simulink model "DV3A_String1_Diode"  (R2023b)
settings: Solver=VariableStepAuto  StartTime=0.0  StopTime=1  FixedStep=Ts_Power  MinStep=0.0025  RelTol=1e-4
PreLoadFcn:
  | Ts_Power=5e-4;
  | Slope_Vdc=1;
InitFcn:
  | Ts_Power=50e-6;
  | Tc=1e-5;%break algebraic loop time constant
StopFcn:
  | if exist('I','var') && exist('V','var')
  |    figure(1)
  |    clf
  |    n=find(I>=0);
  |    n=n(end);
  |    Vglobal=V(1:n);
  |    Iglobal=I(1:n);
  | 
  | 
  |    Pglobal=Vglobal.*Iglobal;
  |    n=find(Pglobal==max(Pglobal));
  |    Pmax=Pglobal(n);
  |    Vmp=Vglobal(n);
  |    Imp=Iglobal(n);
  | 
  | 
  |    subplot(211)
  |    plot(Vglobal, Iglobal,Vmp,Imp,'or')
  |    ylabel('Current (A)')
  |    title(sprintf('Global I-V & P-V characteristics\n %s' ,ModuleName))
  | 
  | 
  |    subplot(212)
  |    plot(Vglobal, Pglobal,Vmp,Pmax,'or')
  |    ylabel('Power (W)')
  |    xlabel('Voltage (V)')
  | end
model workspace (MAT data in the model file):
  slope_Vdc = 3.0848387096
undefined symbols (not defined in the file): Slope_Vdc_string1
libraries: spsPVArrayLib x142, spsVariableResistorLib x142, spsDiodeLib x29, spsCurrentMeasurementLib x1, spsVoltageMeasurementLib x1, spsControlledVoltageSourceLib x1, simulink x1, spspowerguiLib x1
(part 2 of 8)

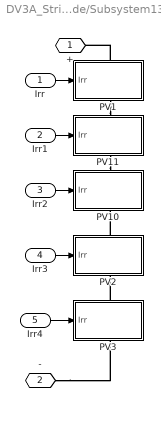
== system DV3A_String1_Diode/Subsystem13 ==
  Irr : Inport
  Irr1 : Inport  Port=2
  Irr2 : Inport  Port=3
  Irr3 : Inport  Port=4
  Irr4 : Inport  Port=5
  PV1 : Subsystem
      settings: PortSchema="{\"entries\":[{\"content\":{\"sides\":[{\"content\":{\"connectorIds\":[\"In1\"]},\"type\":\"ConnectorPlacement.EquallySpacedRectSide\",\"uuid\":\"5c508248-bd07-48d5-951d-be180bcc8740\"},{\"content\":{\"connectorIds\":[],\"side\":\"RIGHT\"},\"type\":\"ConnectorPlacement.EquallySpacedRectSide\",\"uuid\":\"e31a9bdc-b533-497f-8610-a92a4eef02bc\"},{\"content\":{\"connectorIds\":[\"LConn1\"],\"side\":\"TOP\"},\"type\":\"ConnectorPlacement.EquallySpacedRectSide\",\"uuid\":\"a80efd6c-0c74-41ec-a161-3d709011a457\"},{\"content\":{\"connectorIds\":[\"RConn1\"],\"side\":\"BOTTOM\"},\"type\":\"ConnectorPlacement.EquallySpacedRectSide\",\"uuid\":\"e2d028a7-872a-45fc-84e4-cb840db01281\"}]},\"type\":\"ConnectorPlacement.EquallySpacedConnector\",\"uuid\":\"57d442c0-d58c-4dd4-aeba-72d113e063d7\"}],\"packageUris\":[\"http://schema.mathworks.com/mf0/Connector/19700101\"],\"version\":\"1.0\"}"
  PV10 : Subsystem
      settings: PortSchema="{\"entries\":[{\"content\":{\"sides\":[{\"content\":{\"connectorIds\":[\"In1\"]},\"type\":\"ConnectorPlacement.EquallySpacedRectSide\",\"uuid\":\"5c508248-bd07-48d5-951d-be180bcc8740\"},{\"content\":{\"connectorIds\":[],\"side\":\"RIGHT\"},\"type\":\"ConnectorPlacement.EquallySpacedRectSide\",\"uuid\":\"e31a9bdc-b533-497f-8610-a92a4eef02bc\"},{\"content\":{\"connectorIds\":[\"LConn1\"],\"side\":\"TOP\"},\"type\":\"ConnectorPlacement.EquallySpacedRectSide\",\"uuid\":\"a80efd6c-0c74-41ec-a161-3d709011a457\"},{\"content\":{\"connectorIds\":[\"RConn1\"],\"side\":\"BOTTOM\"},\"type\":\"ConnectorPlacement.EquallySpacedRectSide\",\"uuid\":\"e2d028a7-872a-45fc-84e4-cb840db01281\"}]},\"type\":\"ConnectorPlacement.EquallySpacedConnector\",\"uuid\":\"57d442c0-d58c-4dd4-aeba-72d113e063d7\"}],\"packageUris\":[\"http://schema.mathworks.com/mf0/Connector/19700101\"],\"version\":\"1.0\"}"
  PV11 : Subsystem
      settings: PortSchema="{\"entries\":[{\"content\":{\"sides\":[{\"content\":{\"connectorIds\":[\"In1\"]},\"type\":\"ConnectorPlacement.EquallySpacedRectSide\",\"uuid\":\"5c508248-bd07-48d5-951d-be180bcc8740\"},{\"content\":{\"connectorIds\":[],\"side\":\"RIGHT\"},\"type\":\"ConnectorPlacement.EquallySpacedRectSide\",\"uuid\":\"e31a9bdc-b533-497f-8610-a92a4eef02bc\"},{\"content\":{\"connectorIds\":[\"LConn1\"],\"side\":\"TOP\"},\"type\":\"ConnectorPlacement.EquallySpacedRectSide\",\"uuid\":\"a80efd6c-0c74-41ec-a161-3d709011a457\"},{\"content\":{\"connectorIds\":[\"RConn1\"],\"side\":\"BOTTOM\"},\"type\":\"ConnectorPlacement.EquallySpacedRectSide\",\"uuid\":\"e2d028a7-872a-45fc-84e4-cb840db01281\"}]},\"type\":\"ConnectorPlacement.EquallySpacedConnector\",\"uuid\":\"57d442c0-d58c-4dd4-aeba-72d113e063d7\"}],\"packageUris\":[\"http://schema.mathworks.com/mf0/Connector/19700101\"],\"version\":\"1.0\"}"
  PV2 : Subsystem
      settings: PortSchema="{\"entries\":[{\"content\":{\"sides\":[{\"content\":{\"connectorIds\":[\"In1\"]},\"type\":\"ConnectorPlacement.EquallySpacedRectSide\",\"uuid\":\"5c508248-bd07-48d5-951d-be180bcc8740\"},{\"content\":{\"connectorIds\":[],\"side\":\"RIGHT\"},\"type\":\"ConnectorPlacement.EquallySpacedRectSide\",\"uuid\":\"e31a9bdc-b533-497f-8610-a92a4eef02bc\"},{\"content\":{\"connectorIds\":[\"LConn1\"],\"side\":\"TOP\"},\"type\":\"ConnectorPlacement.EquallySpacedRectSide\",\"uuid\":\"a80efd6c-0c74-41ec-a161-3d709011a457\"},{\"content\":{\"connectorIds\":[\"RConn1\"],\"side\":\"BOTTOM\"},\"type\":\"ConnectorPlacement.EquallySpacedRectSide\",\"uuid\":\"e2d028a7-872a-45fc-84e4-cb840db01281\"}]},\"type\":\"ConnectorPlacement.EquallySpacedConnector\",\"uuid\":\"57d442c0-d58c-4dd4-aeba-72d113e063d7\"}],\"packageUris\":[\"http://schema.mathworks.com/mf0/Connector/19700101\"],\"version\":\"1.0\"}"
  PV3 : Subsystem
      settings: PortSchema="{\"entries\":[{\"content\":{\"sides\":[{\"content\":{\"connectorIds\":[\"In1\"]},\"type\":\"ConnectorPlacement.EquallySpacedRectSide\",\"uuid\":\"5c508248-bd07-48d5-951d-be180bcc8740\"},{\"content\":{\"connectorIds\":[],\"side\":\"RIGHT\"},\"type\":\"ConnectorPlacement.EquallySpacedRectSide\",\"uuid\":\"e31a9bdc-b533-497f-8610-a92a4eef02bc\"},{\"content\":{\"connectorIds\":[\"LConn1\"],\"side\":\"TOP\"},\"type\":\"ConnectorPlacement.EquallySpacedRectSide\",\"uuid\":\"a80efd6c-0c74-41ec-a161-3d709011a457\"},{\"content\":{\"connectorIds\":[\"RConn1\"],\"side\":\"BOTTOM\"},\"type\":\"ConnectorPlacement.EquallySpacedRectSide\",\"uuid\":\"e2d028a7-872a-45fc-84e4-cb840db01281\"}]},\"type\":\"ConnectorPlacement.EquallySpacedConnector\",\"uuid\":\"57d442c0-d58c-4dd4-aeba-72d113e063d7\"}],\"packageUris\":[\"http://schema.mathworks.com/mf0/Connector/19700101\"],\"version\":\"1.0\"}"
  + : PMIOPort  Side=Left
  - : PMIOPort  Port=2  Side=Right
  wires:
  Irr2/1 -> PV10/1(Irr)
  Irr/1 -> PV1/1(Irr)
  Irr1/1 -> PV11/1(Irr)
  Irr3/1 -> PV2/1(Irr)
  Irr4/1 -> PV3/1(Irr)
  connections:
  PV1/LConn1 -- +/RConn1
  PV11/RConn1 -- PV10/LConn1
  PV1/RConn1 -- PV11/LConn1
  PV2/LConn1 -- PV10/RConn1
  PV3/LConn1 -- PV2/RConn1
  -/RConn1 -- PV3/RConn1

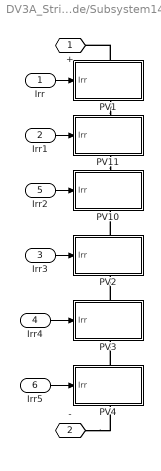
== system DV3A_String1_Diode/Subsystem14 ==
  Irr : Inport
  Irr1 : Inport  Port=2
  Irr3 : Inport  Port=3
  Irr4 : Inport  Port=4
  Irr2 : Inport  Port=5
  Irr5 : Inport  Port=6
  PV1 : Subsystem
      settings: PortSchema="{\"entries\":[{\"content\":{\"sides\":[{\"content\":{\"connectorIds\":[\"In1\"]},\"type\":\"ConnectorPlacement.EquallySpacedRectSide\",\"uuid\":\"5c508248-bd07-48d5-951d-be180bcc8740\"},{\"content\":{\"connectorIds\":[],\"side\":\"RIGHT\"},\"type\":\"ConnectorPlacement.EquallySpacedRectSide\",\"uuid\":\"e31a9bdc-b533-497f-8610-a92a4eef02bc\"},{\"content\":{\"connectorIds\":[\"LConn1\"],\"side\":\"TOP\"},\"type\":\"ConnectorPlacement.EquallySpacedRectSide\",\"uuid\":\"a80efd6c-0c74-41ec-a161-3d709011a457\"},{\"content\":{\"connectorIds\":[\"RConn1\"],\"side\":\"BOTTOM\"},\"type\":\"ConnectorPlacement.EquallySpacedRectSide\",\"uuid\":\"e2d028a7-872a-45fc-84e4-cb840db01281\"}]},\"type\":\"ConnectorPlacement.EquallySpacedConnector\",\"uuid\":\"57d442c0-d58c-4dd4-aeba-72d113e063d7\"}],\"packageUris\":[\"http://schema.mathworks.com/mf0/Connector/19700101\"],\"version\":\"1.0\"}"
  PV10 : Subsystem
      settings: PortSchema="{\"entries\":[{\"content\":{\"sides\":[{\"content\":{\"connectorIds\":[\"In1\"]},\"type\":\"ConnectorPlacement.EquallySpacedRectSide\",\"uuid\":\"5c508248-bd07-48d5-951d-be180bcc8740\"},{\"content\":{\"connectorIds\":[],\"side\":\"RIGHT\"},\"type\":\"ConnectorPlacement.EquallySpacedRectSide\",\"uuid\":\"e31a9bdc-b533-497f-8610-a92a4eef02bc\"},{\"content\":{\"connectorIds\":[\"LConn1\"],\"side\":\"TOP\"},\"type\":\"ConnectorPlacement.EquallySpacedRectSide\",\"uuid\":\"a80efd6c-0c74-41ec-a161-3d709011a457\"},{\"content\":{\"connectorIds\":[\"RConn1\"],\"side\":\"BOTTOM\"},\"type\":\"ConnectorPlacement.EquallySpacedRectSide\",\"uuid\":\"e2d028a7-872a-45fc-84e4-cb840db01281\"}]},\"type\":\"ConnectorPlacement.EquallySpacedConnector\",\"uuid\":\"57d442c0-d58c-4dd4-aeba-72d113e063d7\"}],\"packageUris\":[\"http://schema.mathworks.com/mf0/Connector/19700101\"],\"version\":\"1.0\"}"
  PV11 : Subsystem
      settings: PortSchema="{\"entries\":[{\"content\":{\"sides\":[{\"content\":{\"connectorIds\":[\"In1\"]},\"type\":\"ConnectorPlacement.EquallySpacedRectSide\",\"uuid\":\"5c508248-bd07-48d5-951d-be180bcc8740\"},{\"content\":{\"connectorIds\":[],\"side\":\"RIGHT\"},\"type\":\"ConnectorPlacement.EquallySpacedRectSide\",\"uuid\":\"e31a9bdc-b533-497f-8610-a92a4eef02bc\"},{\"content\":{\"connectorIds\":[\"LConn1\"],\"side\":\"TOP\"},\"type\":\"ConnectorPlacement.EquallySpacedRectSide\",\"uuid\":\"a80efd6c-0c74-41ec-a161-3d709011a457\"},{\"content\":{\"connectorIds\":[\"RConn1\"],\"side\":\"BOTTOM\"},\"type\":\"ConnectorPlacement.EquallySpacedRectSide\",\"uuid\":\"e2d028a7-872a-45fc-84e4-cb840db01281\"}]},\"type\":\"ConnectorPlacement.EquallySpacedConnector\",\"uuid\":\"57d442c0-d58c-4dd4-aeba-72d113e063d7\"}],\"packageUris\":[\"http://schema.mathworks.com/mf0/Connector/19700101\"],\"version\":\"1.0\"}"
  PV2 : Subsystem
      settings: PortSchema="{\"entries\":[{\"content\":{\"sides\":[{\"content\":{\"connectorIds\":[\"In1\"]},\"type\":\"ConnectorPlacement.EquallySpacedRectSide\",\"uuid\":\"5c508248-bd07-48d5-951d-be180bcc8740\"},{\"content\":{\"connectorIds\":[],\"side\":\"RIGHT\"},\"type\":\"ConnectorPlacement.EquallySpacedRectSide\",\"uuid\":\"e31a9bdc-b533-497f-8610-a92a4eef02bc\"},{\"content\":{\"connectorIds\":[\"LConn1\"],\"side\":\"TOP\"},\"type\":\"ConnectorPlacement.EquallySpacedRectSide\",\"uuid\":\"a80efd6c-0c74-41ec-a161-3d709011a457\"},{\"content\":{\"connectorIds\":[\"RConn1\"],\"side\":\"BOTTOM\"},\"type\":\"ConnectorPlacement.EquallySpacedRectSide\",\"uuid\":\"e2d028a7-872a-45fc-84e4-cb840db01281\"}]},\"type\":\"ConnectorPlacement.EquallySpacedConnector\",\"uuid\":\"57d442c0-d58c-4dd4-aeba-72d113e063d7\"}],\"packageUris\":[\"http://schema.mathworks.com/mf0/Connector/19700101\"],\"version\":\"1.0\"}"
  PV3 : Subsystem
      settings: PortSchema="{\"entries\":[{\"content\":{\"sides\":[{\"content\":{\"connectorIds\":[\"In1\"]},\"type\":\"ConnectorPlacement.EquallySpacedRectSide\",\"uuid\":\"5c508248-bd07-48d5-951d-be180bcc8740\"},{\"content\":{\"connectorIds\":[],\"side\":\"RIGHT\"},\"type\":\"ConnectorPlacement.EquallySpacedRectSide\",\"uuid\":\"e31a9bdc-b533-497f-8610-a92a4eef02bc\"},{\"content\":{\"connectorIds\":[\"LConn1\"],\"side\":\"TOP\"},\"type\":\"ConnectorPlacement.EquallySpacedRectSide\",\"uuid\":\"a80efd6c-0c74-41ec-a161-3d709011a457\"},{\"content\":{\"connectorIds\":[\"RConn1\"],\"side\":\"BOTTOM\"},\"type\":\"ConnectorPlacement.EquallySpacedRectSide\",\"uuid\":\"e2d028a7-872a-45fc-84e4-cb840db01281\"}]},\"type\":\"ConnectorPlacement.EquallySpacedConnector\",\"uuid\":\"57d442c0-d58c-4dd4-aeba-72d113e063d7\"}],\"packageUris\":[\"http://schema.mathworks.com/mf0/Connector/19700101\"],\"version\":\"1.0\"}"
  PV4 : Subsystem
      settings: PortSchema="{\"entries\":[{\"content\":{\"sides\":[{\"content\":{\"connectorIds\":[\"In1\"]},\"type\":\"ConnectorPlacement.EquallySpacedRectSide\",\"uuid\":\"5c508248-bd07-48d5-951d-be180bcc8740\"},{\"content\":{\"connectorIds\":[],\"side\":\"RIGHT\"},\"type\":\"ConnectorPlacement.EquallySpacedRectSide\",\"uuid\":\"e31a9bdc-b533-497f-8610-a92a4eef02bc\"},{\"content\":{\"connectorIds\":[\"LConn1\"],\"side\":\"TOP\"},\"type\":\"ConnectorPlacement.EquallySpacedRectSide\",\"uuid\":\"a80efd6c-0c74-41ec-a161-3d709011a457\"},{\"content\":{\"connectorIds\":[\"RConn1\"],\"side\":\"BOTTOM\"},\"type\":\"ConnectorPlacement.EquallySpacedRectSide\",\"uuid\":\"e2d028a7-872a-45fc-84e4-cb840db01281\"}]},\"type\":\"ConnectorPlacement.EquallySpacedConnector\",\"uuid\":\"57d442c0-d58c-4dd4-aeba-72d113e063d7\"}],\"packageUris\":[\"http://schema.mathworks.com/mf0/Connector/19700101\"],\"version\":\"1.0\"}"
  + : PMIOPort  Side=Left
  - : PMIOPort  Port=2  Side=Right
  wires:
  Irr2/1 -> PV10/1(Irr)
  Irr/1 -> PV1/1(Irr)
  Irr1/1 -> PV11/1(Irr)
  Irr3/1 -> PV2/1(Irr)
  Irr4/1 -> PV3/1(Irr)
  Irr5/1 -> PV4/1(Irr)
  connections:
  PV1/LConn1 -- +/RConn1
  PV11/RConn1 -- PV10/LConn1
  PV1/RConn1 -- PV11/LConn1
  PV2/LConn1 -- PV10/RConn1
  PV3/LConn1 -- PV2/RConn1
  PV4/LConn1 -- PV3/RConn1
  -/RConn1 -- PV4/RConn1

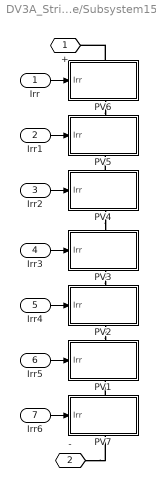
== system DV3A_String1_Diode/Subsystem15 ==
  Irr : Inport
  Irr1 : Inport  Port=2
  Irr2 : Inport  Port=3
  Irr3 : Inport  Port=4
  Irr4 : Inport  Port=5
  Irr5 : Inport  Port=6
  Irr6 : Inport  Port=7
  PV1 : Subsystem
      settings: PortSchema="{\"entries\":[{\"content\":{\"sides\":[{\"content\":{\"connectorIds\":[\"In1\"]},\"type\":\"ConnectorPlacement.EquallySpacedRectSide\",\"uuid\":\"5c508248-bd07-48d5-951d-be180bcc8740\"},{\"content\":{\"connectorIds\":[],\"side\":\"RIGHT\"},\"type\":\"ConnectorPlacement.EquallySpacedRectSide\",\"uuid\":\"e31a9bdc-b533-497f-8610-a92a4eef02bc\"},{\"content\":{\"connectorIds\":[\"LConn1\"],\"side\":\"TOP\"},\"type\":\"ConnectorPlacement.EquallySpacedRectSide\",\"uuid\":\"a80efd6c-0c74-41ec-a161-3d709011a457\"},{\"content\":{\"connectorIds\":[\"RConn1\"],\"side\":\"BOTTOM\"},\"type\":\"ConnectorPlacement.EquallySpacedRectSide\",\"uuid\":\"e2d028a7-872a-45fc-84e4-cb840db01281\"}]},\"type\":\"ConnectorPlacement.EquallySpacedConnector\",\"uuid\":\"57d442c0-d58c-4dd4-aeba-72d113e063d7\"}],\"packageUris\":[\"http://schema.mathworks.com/mf0/Connector/19700101\"],\"version\":\"1.0\"}"
  PV2 : Subsystem
      settings: PortSchema="{\"entries\":[{\"content\":{\"sides\":[{\"content\":{\"connectorIds\":[\"In1\"]},\"type\":\"ConnectorPlacement.EquallySpacedRectSide\",\"uuid\":\"5c508248-bd07-48d5-951d-be180bcc8740\"},{\"content\":{\"connectorIds\":[],\"side\":\"RIGHT\"},\"type\":\"ConnectorPlacement.EquallySpacedRectSide\",\"uuid\":\"e31a9bdc-b533-497f-8610-a92a4eef02bc\"},{\"content\":{\"connectorIds\":[\"LConn1\"],\"side\":\"TOP\"},\"type\":\"ConnectorPlacement.EquallySpacedRectSide\",\"uuid\":\"a80efd6c-0c74-41ec-a161-3d709011a457\"},{\"content\":{\"connectorIds\":[\"RConn1\"],\"side\":\"BOTTOM\"},\"type\":\"ConnectorPlacement.EquallySpacedRectSide\",\"uuid\":\"e2d028a7-872a-45fc-84e4-cb840db01281\"}]},\"type\":\"ConnectorPlacement.EquallySpacedConnector\",\"uuid\":\"57d442c0-d58c-4dd4-aeba-72d113e063d7\"}],\"packageUris\":[\"http://schema.mathworks.com/mf0/Connector/19700101\"],\"version\":\"1.0\"}"
  PV3 : Subsystem
      settings: PortSchema="{\"entries\":[{\"content\":{\"sides\":[{\"content\":{\"connectorIds\":[\"In1\"]},\"type\":\"ConnectorPlacement.EquallySpacedRectSide\",\"uuid\":\"5c508248-bd07-48d5-951d-be180bcc8740\"},{\"content\":{\"connectorIds\":[],\"side\":\"RIGHT\"},\"type\":\"ConnectorPlacement.EquallySpacedRectSide\",\"uuid\":\"e31a9bdc-b533-497f-8610-a92a4eef02bc\"},{\"content\":{\"connectorIds\":[\"LConn1\"],\"side\":\"TOP\"},\"type\":\"ConnectorPlacement.EquallySpacedRectSide\",\"uuid\":\"a80efd6c-0c74-41ec-a161-3d709011a457\"},{\"content\":{\"connectorIds\":[\"RConn1\"],\"side\":\"BOTTOM\"},\"type\":\"ConnectorPlacement.EquallySpacedRectSide\",\"uuid\":\"e2d028a7-872a-45fc-84e4-cb840db01281\"}]},\"type\":\"ConnectorPlacement.EquallySpacedConnector\",\"uuid\":\"57d442c0-d58c-4dd4-aeba-72d113e063d7\"}],\"packageUris\":[\"http://schema.mathworks.com/mf0/Connector/19700101\"],\"version\":\"1.0\"}"
  PV4 : Subsystem
      settings: PortSchema="{\"entries\":[{\"content\":{\"sides\":[{\"content\":{\"connectorIds\":[\"In1\"]},\"type\":\"ConnectorPlacement.EquallySpacedRectSide\",\"uuid\":\"5c508248-bd07-48d5-951d-be180bcc8740\"},{\"content\":{\"connectorIds\":[],\"side\":\"RIGHT\"},\"type\":\"ConnectorPlacement.EquallySpacedRectSide\",\"uuid\":\"e31a9bdc-b533-497f-8610-a92a4eef02bc\"},{\"content\":{\"connectorIds\":[\"LConn1\"],\"side\":\"TOP\"},\"type\":\"ConnectorPlacement.EquallySpacedRectSide\",\"uuid\":\"a80efd6c-0c74-41ec-a161-3d709011a457\"},{\"content\":{\"connectorIds\":[\"RConn1\"],\"side\":\"BOTTOM\"},\"type\":\"ConnectorPlacement.EquallySpacedRectSide\",\"uuid\":\"e2d028a7-872a-45fc-84e4-cb840db01281\"}]},\"type\":\"ConnectorPlacement.EquallySpacedConnector\",\"uuid\":\"57d442c0-d58c-4dd4-aeba-72d113e063d7\"}],\"packageUris\":[\"http://schema.mathworks.com/mf0/Connector/19700101\"],\"version\":\"1.0\"}"
  PV5 : Subsystem
      settings: PortSchema="{\"entries\":[{\"content\":{\"sides\":[{\"content\":{\"connectorIds\":[\"In1\"]},\"type\":\"ConnectorPlacement.EquallySpacedRectSide\",\"uuid\":\"5c508248-bd07-48d5-951d-be180bcc8740\"},{\"content\":{\"connectorIds\":[],\"side\":\"RIGHT\"},\"type\":\"ConnectorPlacement.EquallySpacedRectSide\",\"uuid\":\"e31a9bdc-b533-497f-8610-a92a4eef02bc\"},{\"content\":{\"connectorIds\":[\"LConn1\"],\"side\":\"TOP\"},\"type\":\"ConnectorPlacement.EquallySpacedRectSide\",\"uuid\":\"a80efd6c-0c74-41ec-a161-3d709011a457\"},{\"content\":{\"connectorIds\":[\"RConn1\"],\"side\":\"BOTTOM\"},\"type\":\"ConnectorPlacement.EquallySpacedRectSide\",\"uuid\":\"e2d028a7-872a-45fc-84e4-cb840db01281\"}]},\"type\":\"ConnectorPlacement.EquallySpacedConnector\",\"uuid\":\"57d442c0-d58c-4dd4-aeba-72d113e063d7\"}],\"packageUris\":[\"http://schema.mathworks.com/mf0/Connector/19700101\"],\"version\":\"1.0\"}"
  PV6 : Subsystem
      settings: PortSchema="{\"entries\":[{\"content\":{\"sides\":[{\"content\":{\"connectorIds\":[\"In1\"]},\"type\":\"ConnectorPlacement.EquallySpacedRectSide\",\"uuid\":\"5c508248-bd07-48d5-951d-be180bcc8740\"},{\"content\":{\"connectorIds\":[],\"side\":\"RIGHT\"},\"type\":\"ConnectorPlacement.EquallySpacedRectSide\",\"uuid\":\"e31a9bdc-b533-497f-8610-a92a4eef02bc\"},{\"content\":{\"connectorIds\":[\"LConn1\"],\"side\":\"TOP\"},\"type\":\"ConnectorPlacement.EquallySpacedRectSide\",\"uuid\":\"a80efd6c-0c74-41ec-a161-3d709011a457\"},{\"content\":{\"connectorIds\":[\"RConn1\"],\"side\":\"BOTTOM\"},\"type\":\"ConnectorPlacement.EquallySpacedRectSide\",\"uuid\":\"e2d028a7-872a-45fc-84e4-cb840db01281\"}]},\"type\":\"ConnectorPlacement.EquallySpacedConnector\",\"uuid\":\"57d442c0-d58c-4dd4-aeba-72d113e063d7\"}],\"packageUris\":[\"http://schema.mathworks.com/mf0/Connector/19700101\"],\"version\":\"1.0\"}"
  PV7 : Subsystem
      settings: PortSchema="{\"entries\":[{\"content\":{\"sides\":[{\"content\":{\"connectorIds\":[\"In1\"]},\"type\":\"ConnectorPlacement.EquallySpacedRectSide\",\"uuid\":\"5c508248-bd07-48d5-951d-be180bcc8740\"},{\"content\":{\"connectorIds\":[],\"side\":\"RIGHT\"},\"type\":\"ConnectorPlacement.EquallySpacedRectSide\",\"uuid\":\"e31a9bdc-b533-497f-8610-a92a4eef02bc\"},{\"content\":{\"connectorIds\":[\"LConn1\"],\"side\":\"TOP\"},\"type\":\"ConnectorPlacement.EquallySpacedRectSide\",\"uuid\":\"a80efd6c-0c74-41ec-a161-3d709011a457\"},{\"content\":{\"connectorIds\":[\"RConn1\"],\"side\":\"BOTTOM\"},\"type\":\"ConnectorPlacement.EquallySpacedRectSide\",\"uuid\":\"e2d028a7-872a-45fc-84e4-cb840db01281\"}]},\"type\":\"ConnectorPlacement.EquallySpacedConnector\",\"uuid\":\"57d442c0-d58c-4dd4-aeba-72d113e063d7\"}],\"packageUris\":[\"http://schema.mathworks.com/mf0/Connector/19700101\"],\"version\":\"1.0\"}"
  + : PMIOPort  Side=Left
  - : PMIOPort  Port=2  Side=Right
  wires:
  Irr2/1 -> PV4/1(Irr)
  Irr/1 -> PV6/1(Irr)
  Irr1/1 -> PV5/1(Irr)
  Irr3/1 -> PV3/1(Irr)
  Irr5/1 -> PV1/1(Irr)
  Irr4/1 -> PV2/1(Irr)
  Irr6/1 -> PV7/1(Irr)
  connections:
  PV6/LConn1 -- +/RConn1
  PV4/LConn1 -- PV5/RConn1
  PV6/RConn1 -- PV5/LConn1
  PV3/RConn1 -- PV2/LConn1
  PV2/RConn1 -- PV1/LConn1
  PV4/RConn1 -- PV3/LConn1
  -/RConn1 -- PV7/RConn1
  PV7/LConn1 -- PV1/RConn1

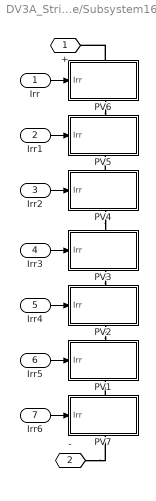
== system DV3A_String1_Diode/Subsystem16 ==
  Irr : Inport
  Irr1 : Inport  Port=2
  Irr2 : Inport  Port=3
  Irr3 : Inport  Port=4
  Irr4 : Inport  Port=5
  Irr5 : Inport  Port=6
  Irr6 : Inport  Port=7
  PV1 : Subsystem
      settings: PortSchema="{\"entries\":[{\"content\":{\"sides\":[{\"content\":{\"connectorIds\":[\"In1\"]},\"type\":\"ConnectorPlacement.EquallySpacedRectSide\",\"uuid\":\"5c508248-bd07-48d5-951d-be180bcc8740\"},{\"content\":{\"connectorIds\":[],\"side\":\"RIGHT\"},\"type\":\"ConnectorPlacement.EquallySpacedRectSide\",\"uuid\":\"e31a9bdc-b533-497f-8610-a92a4eef02bc\"},{\"content\":{\"connectorIds\":[\"LConn1\"],\"side\":\"TOP\"},\"type\":\"ConnectorPlacement.EquallySpacedRectSide\",\"uuid\":\"a80efd6c-0c74-41ec-a161-3d709011a457\"},{\"content\":{\"connectorIds\":[\"RConn1\"],\"side\":\"BOTTOM\"},\"type\":\"ConnectorPlacement.EquallySpacedRectSide\",\"uuid\":\"e2d028a7-872a-45fc-84e4-cb840db01281\"}]},\"type\":\"ConnectorPlacement.EquallySpacedConnector\",\"uuid\":\"57d442c0-d58c-4dd4-aeba-72d113e063d7\"}],\"packageUris\":[\"http://schema.mathworks.com/mf0/Connector/19700101\"],\"version\":\"1.0\"}"
  PV2 : Subsystem
      settings: PortSchema="{\"entries\":[{\"content\":{\"sides\":[{\"content\":{\"connectorIds\":[\"In1\"]},\"type\":\"ConnectorPlacement.EquallySpacedRectSide\",\"uuid\":\"5c508248-bd07-48d5-951d-be180bcc8740\"},{\"content\":{\"connectorIds\":[],\"side\":\"RIGHT\"},\"type\":\"ConnectorPlacement.EquallySpacedRectSide\",\"uuid\":\"e31a9bdc-b533-497f-8610-a92a4eef02bc\"},{\"content\":{\"connectorIds\":[\"LConn1\"],\"side\":\"TOP\"},\"type\":\"ConnectorPlacement.EquallySpacedRectSide\",\"uuid\":\"a80efd6c-0c74-41ec-a161-3d709011a457\"},{\"content\":{\"connectorIds\":[\"RConn1\"],\"side\":\"BOTTOM\"},\"type\":\"ConnectorPlacement.EquallySpacedRectSide\",\"uuid\":\"e2d028a7-872a-45fc-84e4-cb840db01281\"}]},\"type\":\"ConnectorPlacement.EquallySpacedConnector\",\"uuid\":\"57d442c0-d58c-4dd4-aeba-72d113e063d7\"}],\"packageUris\":[\"http://schema.mathworks.com/mf0/Connector/19700101\"],\"version\":\"1.0\"}"
  PV3 : Subsystem
      settings: PortSchema="{\"entries\":[{\"content\":{\"sides\":[{\"content\":{\"connectorIds\":[\"In1\"]},\"type\":\"ConnectorPlacement.EquallySpacedRectSide\",\"uuid\":\"5c508248-bd07-48d5-951d-be180bcc8740\"},{\"content\":{\"connectorIds\":[],\"side\":\"RIGHT\"},\"type\":\"ConnectorPlacement.EquallySpacedRectSide\",\"uuid\":\"e31a9bdc-b533-497f-8610-a92a4eef02bc\"},{\"content\":{\"connectorIds\":[\"LConn1\"],\"side\":\"TOP\"},\"type\":\"ConnectorPlacement.EquallySpacedRectSide\",\"uuid\":\"a80efd6c-0c74-41ec-a161-3d709011a457\"},{\"content\":{\"connectorIds\":[\"RConn1\"],\"side\":\"BOTTOM\"},\"type\":\"ConnectorPlacement.EquallySpacedRectSide\",\"uuid\":\"e2d028a7-872a-45fc-84e4-cb840db01281\"}]},\"type\":\"ConnectorPlacement.EquallySpacedConnector\",\"uuid\":\"57d442c0-d58c-4dd4-aeba-72d113e063d7\"}],\"packageUris\":[\"http://schema.mathworks.com/mf0/Connector/19700101\"],\"version\":\"1.0\"}"
  PV4 : Subsystem
      settings: PortSchema="{\"entries\":[{\"content\":{\"sides\":[{\"content\":{\"connectorIds\":[\"In1\"]},\"type\":\"ConnectorPlacement.EquallySpacedRectSide\",\"uuid\":\"5c508248-bd07-48d5-951d-be180bcc8740\"},{\"content\":{\"connectorIds\":[],\"side\":\"RIGHT\"},\"type\":\"ConnectorPlacement.EquallySpacedRectSide\",\"uuid\":\"e31a9bdc-b533-497f-8610-a92a4eef02bc\"},{\"content\":{\"connectorIds\":[\"LConn1\"],\"side\":\"TOP\"},\"type\":\"ConnectorPlacement.EquallySpacedRectSide\",\"uuid\":\"a80efd6c-0c74-41ec-a161-3d709011a457\"},{\"content\":{\"connectorIds\":[\"RConn1\"],\"side\":\"BOTTOM\"},\"type\":\"ConnectorPlacement.EquallySpacedRectSide\",\"uuid\":\"e2d028a7-872a-45fc-84e4-cb840db01281\"}]},\"type\":\"ConnectorPlacement.EquallySpacedConnector\",\"uuid\":\"57d442c0-d58c-4dd4-aeba-72d113e063d7\"}],\"packageUris\":[\"http://schema.mathworks.com/mf0/Connector/19700101\"],\"version\":\"1.0\"}"
  PV5 : Subsystem
      settings: PortSchema="{\"entries\":[{\"content\":{\"sides\":[{\"content\":{\"connectorIds\":[\"In1\"]},\"type\":\"ConnectorPlacement.EquallySpacedRectSide\",\"uuid\":\"5c508248-bd07-48d5-951d-be180bcc8740\"},{\"content\":{\"connectorIds\":[],\"side\":\"RIGHT\"},\"type\":\"ConnectorPlacement.EquallySpacedRectSide\",\"uuid\":\"e31a9bdc-b533-497f-8610-a92a4eef02bc\"},{\"content\":{\"connectorIds\":[\"LConn1\"],\"side\":\"TOP\"},\"type\":\"ConnectorPlacement.EquallySpacedRectSide\",\"uuid\":\"a80efd6c-0c74-41ec-a161-3d709011a457\"},{\"content\":{\"connectorIds\":[\"RConn1\"],\"side\":\"BOTTOM\"},\"type\":\"ConnectorPlacement.EquallySpacedRectSide\",\"uuid\":\"e2d028a7-872a-45fc-84e4-cb840db01281\"}]},\"type\":\"ConnectorPlacement.EquallySpacedConnector\",\"uuid\":\"57d442c0-d58c-4dd4-aeba-72d113e063d7\"}],\"packageUris\":[\"http://schema.mathworks.com/mf0/Connector/19700101\"],\"version\":\"1.0\"}"
  PV6 : Subsystem
      settings: PortSchema="{\"entries\":[{\"content\":{\"sides\":[{\"content\":{\"connectorIds\":[\"In1\"]},\"type\":\"ConnectorPlacement.EquallySpacedRectSide\",\"uuid\":\"5c508248-bd07-48d5-951d-be180bcc8740\"},{\"content\":{\"connectorIds\":[],\"side\":\"RIGHT\"},\"type\":\"ConnectorPlacement.EquallySpacedRectSide\",\"uuid\":\"e31a9bdc-b533-497f-8610-a92a4eef02bc\"},{\"content\":{\"connectorIds\":[\"LConn1\"],\"side\":\"TOP\"},\"type\":\"ConnectorPlacement.EquallySpacedRectSide\",\"uuid\":\"a80efd6c-0c74-41ec-a161-3d709011a457\"},{\"content\":{\"connectorIds\":[\"RConn1\"],\"side\":\"BOTTOM\"},\"type\":\"ConnectorPlacement.EquallySpacedRectSide\",\"uuid\":\"e2d028a7-872a-45fc-84e4-cb840db01281\"}]},\"type\":\"ConnectorPlacement.EquallySpacedConnector\",\"uuid\":\"57d442c0-d58c-4dd4-aeba-72d113e063d7\"}],\"packageUris\":[\"http://schema.mathworks.com/mf0/Connector/19700101\"],\"version\":\"1.0\"}"
  PV7 : Subsystem
      settings: PortSchema="{\"entries\":[{\"content\":{\"sides\":[{\"content\":{\"connectorIds\":[\"In1\"]},\"type\":\"ConnectorPlacement.EquallySpacedRectSide\",\"uuid\":\"5c508248-bd07-48d5-951d-be180bcc8740\"},{\"content\":{\"connectorIds\":[],\"side\":\"RIGHT\"},\"type\":\"ConnectorPlacement.EquallySpacedRectSide\",\"uuid\":\"e31a9bdc-b533-497f-8610-a92a4eef02bc\"},{\"content\":{\"connectorIds\":[\"LConn1\"],\"side\":\"TOP\"},\"type\":\"ConnectorPlacement.EquallySpacedRectSide\",\"uuid\":\"a80efd6c-0c74-41ec-a161-3d709011a457\"},{\"content\":{\"connectorIds\":[\"RConn1\"],\"side\":\"BOTTOM\"},\"type\":\"ConnectorPlacement.EquallySpacedRectSide\",\"uuid\":\"e2d028a7-872a-45fc-84e4-cb840db01281\"}]},\"type\":\"ConnectorPlacement.EquallySpacedConnector\",\"uuid\":\"57d442c0-d58c-4dd4-aeba-72d113e063d7\"}],\"packageUris\":[\"http://schema.mathworks.com/mf0/Connector/19700101\"],\"version\":\"1.0\"}"
  + : PMIOPort  Side=Left
  - : PMIOPort  Port=2  Side=Right
  wires:
  Irr2/1 -> PV4/1(Irr)
  Irr/1 -> PV6/1(Irr)
  Irr1/1 -> PV5/1(Irr)
  Irr3/1 -> PV3/1(Irr)
  Irr5/1 -> PV1/1(Irr)
  Irr4/1 -> PV2/1(Irr)
  Irr6/1 -> PV7/1(Irr)
  connections:
  PV6/LConn1 -- +/RConn1
  PV4/LConn1 -- PV5/RConn1
  PV6/RConn1 -- PV5/LConn1
  PV3/RConn1 -- PV2/LConn1
  PV2/RConn1 -- PV1/LConn1
  PV4/RConn1 -- PV3/LConn1
  -/RConn1 -- PV7/RConn1
  PV7/LConn1 -- PV1/RConn1

== system DV3A_String1_Diode/Subsystem17 ==
  Irr : Inport
  Irr1 : Inport  Port=2
  Irr2 : Inport  Port=3
  Irr3 : Inport  Port=4
  PV1 : Subsystem
      settings: PortSchema="{\"entries\":[{\"content\":{\"sides\":[{\"content\":{\"connectorIds\":[\"In1\"]},\"type\":\"ConnectorPlacement.EquallySpacedRectSide\",\"uuid\":\"5c508248-bd07-48d5-951d-be180bcc8740\"},{\"content\":{\"connectorIds\":[],\"side\":\"RIGHT\"},\"type\":\"ConnectorPlacement.EquallySpacedRectSide\",\"uuid\":\"e31a9bdc-b533-497f-8610-a92a4eef02bc\"},{\"content\":{\"connectorIds\":[\"LConn1\"],\"side\":\"TOP\"},\"type\":\"ConnectorPlacement.EquallySpacedRectSide\",\"uuid\":\"a80efd6c-0c74-41ec-a161-3d709011a457\"},{\"content\":{\"connectorIds\":[\"RConn1\"],\"side\":\"BOTTOM\"},\"type\":\"ConnectorPlacement.EquallySpacedRectSide\",\"uuid\":\"e2d028a7-872a-45fc-84e4-cb840db01281\"}]},\"type\":\"ConnectorPlacement.EquallySpacedConnector\",\"uuid\":\"57d442c0-d58c-4dd4-aeba-72d113e063d7\"}],\"packageUris\":[\"http://schema.mathworks.com/mf0/Connector/19700101\"],\"version\":\"1.0\"}"
  PV2 : Subsystem
      settings: PortSchema="{\"entries\":[{\"content\":{\"sides\":[{\"content\":{\"connectorIds\":[\"In1\"]},\"type\":\"ConnectorPlacement.EquallySpacedRectSide\",\"uuid\":\"5c508248-bd07-48d5-951d-be180bcc8740\"},{\"content\":{\"connectorIds\":[],\"side\":\"RIGHT\"},\"type\":\"ConnectorPlacement.EquallySpacedRectSide\",\"uuid\":\"e31a9bdc-b533-497f-8610-a92a4eef02bc\"},{\"content\":{\"connectorIds\":[\"LConn1\"],\"side\":\"TOP\"},\"type\":\"ConnectorPlacement.EquallySpacedRectSide\",\"uuid\":\"a80efd6c-0c74-41ec-a161-3d709011a457\"},{\"content\":{\"connectorIds\":[\"RConn1\"],\"side\":\"BOTTOM\"},\"type\":\"ConnectorPlacement.EquallySpacedRectSide\",\"uuid\":\"e2d028a7-872a-45fc-84e4-cb840db01281\"}]},\"type\":\"ConnectorPlacement.EquallySpacedConnector\",\"uuid\":\"57d442c0-d58c-4dd4-aeba-72d113e063d7\"}],\"packageUris\":[\"http://schema.mathworks.com/mf0/Connector/19700101\"],\"version\":\"1.0\"}"
  PV3 : Subsystem
      settings: PortSchema="{\"entries\":[{\"content\":{\"sides\":[{\"content\":{\"connectorIds\":[\"In1\"]},\"type\":\"ConnectorPlacement.EquallySpacedRectSide\",\"uuid\":\"5c508248-bd07-48d5-951d-be180bcc8740\"},{\"content\":{\"connectorIds\":[],\"side\":\"RIGHT\"},\"type\":\"ConnectorPlacement.EquallySpacedRectSide\",\"uuid\":\"e31a9bdc-b533-497f-8610-a92a4eef02bc\"},{\"content\":{\"connectorIds\":[\"LConn1\"],\"side\":\"TOP\"},\"type\":\"ConnectorPlacement.EquallySpacedRectSide\",\"uuid\":\"a80efd6c-0c74-41ec-a161-3d709011a457\"},{\"content\":{\"connectorIds\":[\"RConn1\"],\"side\":\"BOTTOM\"},\"type\":\"ConnectorPlacement.EquallySpacedRectSide\",\"uuid\":\"e2d028a7-872a-45fc-84e4-cb840db01281\"}]},\"type\":\"ConnectorPlacement.EquallySpacedConnector\",\"uuid\":\"57d442c0-d58c-4dd4-aeba-72d113e063d7\"}],\"packageUris\":[\"http://schema.mathworks.com/mf0/Connector/19700101\"],\"version\":\"1.0\"}"
  PV4 : Subsystem
      settings: PortSchema="{\"entries\":[{\"content\":{\"sides\":[{\"content\":{\"connectorIds\":[\"In1\"]},\"type\":\"ConnectorPlacement.EquallySpacedRectSide\",\"uuid\":\"5c508248-bd07-48d5-951d-be180bcc8740\"},{\"content\":{\"connectorIds\":[],\"side\":\"RIGHT\"},\"type\":\"ConnectorPlacement.EquallySpacedRectSide\",\"uuid\":\"e31a9bdc-b533-497f-8610-a92a4eef02bc\"},{\"content\":{\"connectorIds\":[\"LConn1\"],\"side\":\"TOP\"},\"type\":\"ConnectorPlacement.EquallySpacedRectSide\",\"uuid\":\"a80efd6c-0c74-41ec-a161-3d709011a457\"},{\"content\":{\"connectorIds\":[\"RConn1\"],\"side\":\"BOTTOM\"},\"type\":\"ConnectorPlacement.EquallySpacedRectSide\",\"uuid\":\"e2d028a7-872a-45fc-84e4-cb840db01281\"}]},\"type\":\"ConnectorPlacement.EquallySpacedConnector\",\"uuid\":\"57d442c0-d58c-4dd4-aeba-72d113e063d7\"}],\"packageUris\":[\"http://schema.mathworks.com/mf0/Connector/19700101\"],\"version\":\"1.0\"}"
  + : PMIOPort  Side=Left
  - : PMIOPort  Port=2  Side=Right
  wires:
  Irr2/1 -> PV1/1(Irr)
  Irr/1 -> PV2/1(Irr)
  Irr1/1 -> PV4/1(Irr)
  Irr3/1 -> PV3/1(Irr)
  connections:
  PV2/LConn1 -- +/RConn1
  PV4/RConn1 -- PV1/LConn1
  PV4/LConn1 -- PV2/RConn1
  PV3/RConn1 -- -/RConn1
  PV1/RConn1 -- PV3/LConn1

== system DV3A_String1_Diode/Subsystem18 ==
  Irr : Inport
  Irr1 : Inport  Port=2
  Irr2 : Inport  Port=3
  Irr3 : Inport  Port=4
  PV1 : Subsystem
      settings: PortSchema="{\"entries\":[{\"content\":{\"sides\":[{\"content\":{\"connectorIds\":[\"In1\"]},\"type\":\"ConnectorPlacement.EquallySpacedRectSide\",\"uuid\":\"5c508248-bd07-48d5-951d-be180bcc8740\"},{\"content\":{\"connectorIds\":[],\"side\":\"RIGHT\"},\"type\":\"ConnectorPlacement.EquallySpacedRectSide\",\"uuid\":\"e31a9bdc-b533-497f-8610-a92a4eef02bc\"},{\"content\":{\"connectorIds\":[\"LConn1\"],\"side\":\"TOP\"},\"type\":\"ConnectorPlacement.EquallySpacedRectSide\",\"uuid\":\"a80efd6c-0c74-41ec-a161-3d709011a457\"},{\"content\":{\"connectorIds\":[\"RConn1\"],\"side\":\"BOTTOM\"},\"type\":\"ConnectorPlacement.EquallySpacedRectSide\",\"uuid\":\"e2d028a7-872a-45fc-84e4-cb840db01281\"}]},\"type\":\"ConnectorPlacement.EquallySpacedConnector\",\"uuid\":\"57d442c0-d58c-4dd4-aeba-72d113e063d7\"}],\"packageUris\":[\"http://schema.mathworks.com/mf0/Connector/19700101\"],\"version\":\"1.0\"}"
  PV2 : Subsystem
      settings: PortSchema="{\"entries\":[{\"content\":{\"sides\":[{\"content\":{\"connectorIds\":[\"In1\"]},\"type\":\"ConnectorPlacement.EquallySpacedRectSide\",\"uuid\":\"5c508248-bd07-48d5-951d-be180bcc8740\"},{\"content\":{\"connectorIds\":[],\"side\":\"RIGHT\"},\"type\":\"ConnectorPlacement.EquallySpacedRectSide\",\"uuid\":\"e31a9bdc-b533-497f-8610-a92a4eef02bc\"},{\"content\":{\"connectorIds\":[\"LConn1\"],\"side\":\"TOP\"},\"type\":\"ConnectorPlacement.EquallySpacedRectSide\",\"uuid\":\"a80efd6c-0c74-41ec-a161-3d709011a457\"},{\"content\":{\"connectorIds\":[\"RConn1\"],\"side\":\"BOTTOM\"},\"type\":\"ConnectorPlacement.EquallySpacedRectSide\",\"uuid\":\"e2d028a7-872a-45fc-84e4-cb840db01281\"}]},\"type\":\"ConnectorPlacement.EquallySpacedConnector\",\"uuid\":\"57d442c0-d58c-4dd4-aeba-72d113e063d7\"}],\"packageUris\":[\"http://schema.mathworks.com/mf0/Connector/19700101\"],\"version\":\"1.0\"}"
  PV3 : Subsystem
      settings: PortSchema="{\"entries\":[{\"content\":{\"sides\":[{\"content\":{\"connectorIds\":[\"In1\"]},\"type\":\"ConnectorPlacement.EquallySpacedRectSide\",\"uuid\":\"5c508248-bd07-48d5-951d-be180bcc8740\"},{\"content\":{\"connectorIds\":[],\"side\":\"RIGHT\"},\"type\":\"ConnectorPlacement.EquallySpacedRectSide\",\"uuid\":\"e31a9bdc-b533-497f-8610-a92a4eef02bc\"},{\"content\":{\"connectorIds\":[\"LConn1\"],\"side\":\"TOP\"},\"type\":\"ConnectorPlacement.EquallySpacedRectSide\",\"uuid\":\"a80efd6c-0c74-41ec-a161-3d709011a457\"},{\"content\":{\"connectorIds\":[\"RConn1\"],\"side\":\"BOTTOM\"},\"type\":\"ConnectorPlacement.EquallySpacedRectSide\",\"uuid\":\"e2d028a7-872a-45fc-84e4-cb840db01281\"}]},\"type\":\"ConnectorPlacement.EquallySpacedConnector\",\"uuid\":\"57d442c0-d58c-4dd4-aeba-72d113e063d7\"}],\"packageUris\":[\"http://schema.mathworks.com/mf0/Connector/19700101\"],\"version\":\"1.0\"}"
  PV4 : Subsystem
      settings: PortSchema="{\"entries\":[{\"content\":{\"sides\":[{\"content\":{\"connectorIds\":[\"In1\"]},\"type\":\"ConnectorPlacement.EquallySpacedRectSide\",\"uuid\":\"5c508248-bd07-48d5-951d-be180bcc8740\"},{\"content\":{\"connectorIds\":[],\"side\":\"RIGHT\"},\"type\":\"ConnectorPlacement.EquallySpacedRectSide\",\"uuid\":\"e31a9bdc-b533-497f-8610-a92a4eef02bc\"},{\"content\":{\"connectorIds\":[\"LConn1\"],\"side\":\"TOP\"},\"type\":\"ConnectorPlacement.EquallySpacedRectSide\",\"uuid\":\"a80efd6c-0c74-41ec-a161-3d709011a457\"},{\"content\":{\"connectorIds\":[\"RConn1\"],\"side\":\"BOTTOM\"},\"type\":\"ConnectorPlacement.EquallySpacedRectSide\",\"uuid\":\"e2d028a7-872a-45fc-84e4-cb840db01281\"}]},\"type\":\"ConnectorPlacement.EquallySpacedConnector\",\"uuid\":\"57d442c0-d58c-4dd4-aeba-72d113e063d7\"}],\"packageUris\":[\"http://schema.mathworks.com/mf0/Connector/19700101\"],\"version\":\"1.0\"}"
  + : PMIOPort  Side=Left
  - : PMIOPort  Port=2  Side=Right
  wires:
  Irr2/1 -> PV1/1(Irr)
  Irr/1 -> PV2/1(Irr)
  Irr1/1 -> PV4/1(Irr)
  Irr3/1 -> PV3/1(Irr)
  connections:
  PV2/LConn1 -- +/RConn1
  PV4/RConn1 -- PV1/LConn1
  PV4/LConn1 -- PV2/RConn1
  PV3/RConn1 -- -/RConn1
  PV1/RConn1 -- PV3/LConn1

== system DV3A_String1_Diode/Subsystem19 ==
  Irr : Inport
  Irr1 : Inport  Port=2
  Irr2 : Inport  Port=3
  Irr3 : Inport  Port=4
  PV1 : Subsystem
      settings: PortSchema="{\"entries\":[{\"content\":{\"sides\":[{\"content\":{\"connectorIds\":[\"In1\"]},\"type\":\"ConnectorPlacement.EquallySpacedRectSide\",\"uuid\":\"5c508248-bd07-48d5-951d-be180bcc8740\"},{\"content\":{\"connectorIds\":[],\"side\":\"RIGHT\"},\"type\":\"ConnectorPlacement.EquallySpacedRectSide\",\"uuid\":\"e31a9bdc-b533-497f-8610-a92a4eef02bc\"},{\"content\":{\"connectorIds\":[\"LConn1\"],\"side\":\"TOP\"},\"type\":\"ConnectorPlacement.EquallySpacedRectSide\",\"uuid\":\"a80efd6c-0c74-41ec-a161-3d709011a457\"},{\"content\":{\"connectorIds\":[\"RConn1\"],\"side\":\"BOTTOM\"},\"type\":\"ConnectorPlacement.EquallySpacedRectSide\",\"uuid\":\"e2d028a7-872a-45fc-84e4-cb840db01281\"}]},\"type\":\"ConnectorPlacement.EquallySpacedConnector\",\"uuid\":\"57d442c0-d58c-4dd4-aeba-72d113e063d7\"}],\"packageUris\":[\"http://schema.mathworks.com/mf0/Connector/19700101\"],\"version\":\"1.0\"}"
  PV2 : Subsystem
      settings: PortSchema="{\"entries\":[{\"content\":{\"sides\":[{\"content\":{\"connectorIds\":[\"In1\"]},\"type\":\"ConnectorPlacement.EquallySpacedRectSide\",\"uuid\":\"5c508248-bd07-48d5-951d-be180bcc8740\"},{\"content\":{\"connectorIds\":[],\"side\":\"RIGHT\"},\"type\":\"ConnectorPlacement.EquallySpacedRectSide\",\"uuid\":\"e31a9bdc-b533-497f-8610-a92a4eef02bc\"},{\"content\":{\"connectorIds\":[\"LConn1\"],\"side\":\"TOP\"},\"type\":\"ConnectorPlacement.EquallySpacedRectSide\",\"uuid\":\"a80efd6c-0c74-41ec-a161-3d709011a457\"},{\"content\":{\"connectorIds\":[\"RConn1\"],\"side\":\"BOTTOM\"},\"type\":\"ConnectorPlacement.EquallySpacedRectSide\",\"uuid\":\"e2d028a7-872a-45fc-84e4-cb840db01281\"}]},\"type\":\"ConnectorPlacement.EquallySpacedConnector\",\"uuid\":\"57d442c0-d58c-4dd4-aeba-72d113e063d7\"}],\"packageUris\":[\"http://schema.mathworks.com/mf0/Connector/19700101\"],\"version\":\"1.0\"}"
  PV3 : Subsystem
      settings: PortSchema="{\"entries\":[{\"content\":{\"sides\":[{\"content\":{\"connectorIds\":[\"In1\"]},\"type\":\"ConnectorPlacement.EquallySpacedRectSide\",\"uuid\":\"5c508248-bd07-48d5-951d-be180bcc8740\"},{\"content\":{\"connectorIds\":[],\"side\":\"RIGHT\"},\"type\":\"ConnectorPlacement.EquallySpacedRectSide\",\"uuid\":\"e31a9bdc-b533-497f-8610-a92a4eef02bc\"},{\"content\":{\"connectorIds\":[\"LConn1\"],\"side\":\"TOP\"},\"type\":\"ConnectorPlacement.EquallySpacedRectSide\",\"uuid\":\"a80efd6c-0c74-41ec-a161-3d709011a457\"},{\"content\":{\"connectorIds\":[\"RConn1\"],\"side\":\"BOTTOM\"},\"type\":\"ConnectorPlacement.EquallySpacedRectSide\",\"uuid\":\"e2d028a7-872a-45fc-84e4-cb840db01281\"}]},\"type\":\"ConnectorPlacement.EquallySpacedConnector\",\"uuid\":\"57d442c0-d58c-4dd4-aeba-72d113e063d7\"}],\"packageUris\":[\"http://schema.mathworks.com/mf0/Connector/19700101\"],\"version\":\"1.0\"}"
  PV4 : Subsystem
      settings: PortSchema="{\"entries\":[{\"content\":{\"sides\":[{\"content\":{\"connectorIds\":[\"In1\"]},\"type\":\"ConnectorPlacement.EquallySpacedRectSide\",\"uuid\":\"5c508248-bd07-48d5-951d-be180bcc8740\"},{\"content\":{\"connectorIds\":[],\"side\":\"RIGHT\"},\"type\":\"ConnectorPlacement.EquallySpacedRectSide\",\"uuid\":\"e31a9bdc-b533-497f-8610-a92a4eef02bc\"},{\"content\":{\"connectorIds\":[\"LConn1\"],\"side\":\"TOP\"},\"type\":\"ConnectorPlacement.EquallySpacedRectSide\",\"uuid\":\"a80efd6c-0c74-41ec-a161-3d709011a457\"},{\"content\":{\"connectorIds\":[\"RConn1\"],\"side\":\"BOTTOM\"},\"type\":\"ConnectorPlacement.EquallySpacedRectSide\",\"uuid\":\"e2d028a7-872a-45fc-84e4-cb840db01281\"}]},\"type\":\"ConnectorPlacement.EquallySpacedConnector\",\"uuid\":\"57d442c0-d58c-4dd4-aeba-72d113e063d7\"}],\"packageUris\":[\"http://schema.mathworks.com/mf0/Connector/19700101\"],\"version\":\"1.0\"}"
  + : PMIOPort  Side=Left
  - : PMIOPort  Port=2  Side=Right
  wires:
  Irr2/1 -> PV1/1(Irr)
  Irr/1 -> PV2/1(Irr)
  Irr1/1 -> PV4/1(Irr)
  Irr3/1 -> PV3/1(Irr)
  connections:
  PV2/LConn1 -- +/RConn1
  PV4/RConn1 -- PV1/LConn1
  PV4/LConn1 -- PV2/RConn1
  PV3/RConn1 -- -/RConn1
  PV1/RConn1 -- PV3/LConn1

== system DV3A_String1_Diode/Subsystem20 ==
  Irr : Inport
  Irr1 : Inport  Port=2
  Irr2 : Inport  Port=3
  Irr3 : Inport  Port=4
  PV1 : Subsystem
      settings: PortSchema="{\"entries\":[{\"content\":{\"sides\":[{\"content\":{\"connectorIds\":[\"In1\"]},\"type\":\"ConnectorPlacement.EquallySpacedRectSide\",\"uuid\":\"5c508248-bd07-48d5-951d-be180bcc8740\"},{\"content\":{\"connectorIds\":[],\"side\":\"RIGHT\"},\"type\":\"ConnectorPlacement.EquallySpacedRectSide\",\"uuid\":\"e31a9bdc-b533-497f-8610-a92a4eef02bc\"},{\"content\":{\"connectorIds\":[\"LConn1\"],\"side\":\"TOP\"},\"type\":\"ConnectorPlacement.EquallySpacedRectSide\",\"uuid\":\"a80efd6c-0c74-41ec-a161-3d709011a457\"},{\"content\":{\"connectorIds\":[\"RConn1\"],\"side\":\"BOTTOM\"},\"type\":\"ConnectorPlacement.EquallySpacedRectSide\",\"uuid\":\"e2d028a7-872a-45fc-84e4-cb840db01281\"}]},\"type\":\"ConnectorPlacement.EquallySpacedConnector\",\"uuid\":\"57d442c0-d58c-4dd4-aeba-72d113e063d7\"}],\"packageUris\":[\"http://schema.mathworks.com/mf0/Connector/19700101\"],\"version\":\"1.0\"}"
  PV2 : Subsystem
      settings: PortSchema="{\"entries\":[{\"content\":{\"sides\":[{\"content\":{\"connectorIds\":[\"In1\"]},\"type\":\"ConnectorPlacement.EquallySpacedRectSide\",\"uuid\":\"5c508248-bd07-48d5-951d-be180bcc8740\"},{\"content\":{\"connectorIds\":[],\"side\":\"RIGHT\"},\"type\":\"ConnectorPlacement.EquallySpacedRectSide\",\"uuid\":\"e31a9bdc-b533-497f-8610-a92a4eef02bc\"},{\"content\":{\"connectorIds\":[\"LConn1\"],\"side\":\"TOP\"},\"type\":\"ConnectorPlacement.EquallySpacedRectSide\",\"uuid\":\"a80efd6c-0c74-41ec-a161-3d709011a457\"},{\"content\":{\"connectorIds\":[\"RConn1\"],\"side\":\"BOTTOM\"},\"type\":\"ConnectorPlacement.EquallySpacedRectSide\",\"uuid\":\"e2d028a7-872a-45fc-84e4-cb840db01281\"}]},\"type\":\"ConnectorPlacement.EquallySpacedConnector\",\"uuid\":\"57d442c0-d58c-4dd4-aeba-72d113e063d7\"}],\"packageUris\":[\"http://schema.mathworks.com/mf0/Connector/19700101\"],\"version\":\"1.0\"}"
  PV3 : Subsystem
      settings: PortSchema="{\"entries\":[{\"content\":{\"sides\":[{\"content\":{\"connectorIds\":[\"In1\"]},\"type\":\"ConnectorPlacement.EquallySpacedRectSide\",\"uuid\":\"5c508248-bd07-48d5-951d-be180bcc8740\"},{\"content\":{\"connectorIds\":[],\"side\":\"RIGHT\"},\"type\":\"ConnectorPlacement.EquallySpacedRectSide\",\"uuid\":\"e31a9bdc-b533-497f-8610-a92a4eef02bc\"},{\"content\":{\"connectorIds\":[\"LConn1\"],\"side\":\"TOP\"},\"type\":\"ConnectorPlacement.EquallySpacedRectSide\",\"uuid\":\"a80efd6c-0c74-41ec-a161-3d709011a457\"},{\"content\":{\"connectorIds\":[\"RConn1\"],\"side\":\"BOTTOM\"},\"type\":\"ConnectorPlacement.EquallySpacedRectSide\",\"uuid\":\"e2d028a7-872a-45fc-84e4-cb840db01281\"}]},\"type\":\"ConnectorPlacement.EquallySpacedConnector\",\"uuid\":\"57d442c0-d58c-4dd4-aeba-72d113e063d7\"}],\"packageUris\":[\"http://schema.mathworks.com/mf0/Connector/19700101\"],\"version\":\"1.0\"}"
  PV4 : Subsystem
      settings: PortSchema="{\"entries\":[{\"content\":{\"sides\":[{\"content\":{\"connectorIds\":[\"In1\"]},\"type\":\"ConnectorPlacement.EquallySpacedRectSide\",\"uuid\":\"5c508248-bd07-48d5-951d-be180bcc8740\"},{\"content\":{\"connectorIds\":[],\"side\":\"RIGHT\"},\"type\":\"ConnectorPlacement.EquallySpacedRectSide\",\"uuid\":\"e31a9bdc-b533-497f-8610-a92a4eef02bc\"},{\"content\":{\"connectorIds\":[\"LConn1\"],\"side\":\"TOP\"},\"type\":\"ConnectorPlacement.EquallySpacedRectSide\",\"uuid\":\"a80efd6c-0c74-41ec-a161-3d709011a457\"},{\"content\":{\"connectorIds\":[\"RConn1\"],\"side\":\"BOTTOM\"},\"type\":\"ConnectorPlacement.EquallySpacedRectSide\",\"uuid\":\"e2d028a7-872a-45fc-84e4-cb840db01281\"}]},\"type\":\"ConnectorPlacement.EquallySpacedConnector\",\"uuid\":\"57d442c0-d58c-4dd4-aeba-72d113e063d7\"}],\"packageUris\":[\"http://schema.mathworks.com/mf0/Connector/19700101\"],\"version\":\"1.0\"}"
  + : PMIOPort  Side=Left
  - : PMIOPort  Port=2  Side=Right
  wires:
  Irr2/1 -> PV1/1(Irr)
  Irr/1 -> PV2/1(Irr)
  Irr1/1 -> PV4/1(Irr)
  Irr3/1 -> PV3/1(Irr)
  connections:
  PV2/LConn1 -- +/RConn1
  PV4/RConn1 -- PV1/LConn1
  PV4/LConn1 -- PV2/RConn1
  PV3/RConn1 -- -/RConn1
  PV1/RConn1 -- PV3/LConn1

== system DV3A_String1_Diode/Subsystem34 ==
  Irr : Inport
  Irr1 : Inport  Port=2
  Irr2 : Inport  Port=3
  Irr3 : Inport  Port=4
  PV1 : Subsystem
      settings: PortSchema="{\"entries\":[{\"content\":{\"sides\":[{\"content\":{\"connectorIds\":[\"In1\"]},\"type\":\"ConnectorPlacement.EquallySpacedRectSide\",\"uuid\":\"5c508248-bd07-48d5-951d-be180bcc8740\"},{\"content\":{\"connectorIds\":[],\"side\":\"RIGHT\"},\"type\":\"ConnectorPlacement.EquallySpacedRectSide\",\"uuid\":\"e31a9bdc-b533-497f-8610-a92a4eef02bc\"},{\"content\":{\"connectorIds\":[\"LConn1\"],\"side\":\"TOP\"},\"type\":\"ConnectorPlacement.EquallySpacedRectSide\",\"uuid\":\"a80efd6c-0c74-41ec-a161-3d709011a457\"},{\"content\":{\"connectorIds\":[\"RConn1\"],\"side\":\"BOTTOM\"},\"type\":\"ConnectorPlacement.EquallySpacedRectSide\",\"uuid\":\"e2d028a7-872a-45fc-84e4-cb840db01281\"}]},\"type\":\"ConnectorPlacement.EquallySpacedConnector\",\"uuid\":\"57d442c0-d58c-4dd4-aeba-72d113e063d7\"}],\"packageUris\":[\"http://schema.mathworks.com/mf0/Connector/19700101\"],\"version\":\"1.0\"}"
  PV2 : Subsystem
      settings: PortSchema="{\"entries\":[{\"content\":{\"sides\":[{\"content\":{\"connectorIds\":[\"In1\"]},\"type\":\"ConnectorPlacement.EquallySpacedRectSide\",\"uuid\":\"5c508248-bd07-48d5-951d-be180bcc8740\"},{\"content\":{\"connectorIds\":[],\"side\":\"RIGHT\"},\"type\":\"ConnectorPlacement.EquallySpacedRectSide\",\"uuid\":\"e31a9bdc-b533-497f-8610-a92a4eef02bc\"},{\"content\":{\"connectorIds\":[\"LConn1\"],\"side\":\"TOP\"},\"type\":\"ConnectorPlacement.EquallySpacedRectSide\",\"uuid\":\"a80efd6c-0c74-41ec-a161-3d709011a457\"},{\"content\":{\"connectorIds\":[\"RConn1\"],\"side\":\"BOTTOM\"},\"type\":\"ConnectorPlacement.EquallySpacedRectSide\",\"uuid\":\"e2d028a7-872a-45fc-84e4-cb840db01281\"}]},\"type\":\"ConnectorPlacement.EquallySpacedConnector\",\"uuid\":\"57d442c0-d58c-4dd4-aeba-72d113e063d7\"}],\"packageUris\":[\"http://schema.mathworks.com/mf0/Connector/19700101\"],\"version\":\"1.0\"}"
  PV3 : Subsystem
      settings: PortSchema="{\"entries\":[{\"content\":{\"sides\":[{\"content\":{\"connectorIds\":[\"In1\"]},\"type\":\"ConnectorPlacement.EquallySpacedRectSide\",\"uuid\":\"5c508248-bd07-48d5-951d-be180bcc8740\"},{\"content\":{\"connectorIds\":[],\"side\":\"RIGHT\"},\"type\":\"ConnectorPlacement.EquallySpacedRectSide\",\"uuid\":\"e31a9bdc-b533-497f-8610-a92a4eef02bc\"},{\"content\":{\"connectorIds\":[\"LConn1\"],\"side\":\"TOP\"},\"type\":\"ConnectorPlacement.EquallySpacedRectSide\",\"uuid\":\"a80efd6c-0c74-41ec-a161-3d709011a457\"},{\"content\":{\"connectorIds\":[\"RConn1\"],\"side\":\"BOTTOM\"},\"type\":\"ConnectorPlacement.EquallySpacedRectSide\",\"uuid\":\"e2d028a7-872a-45fc-84e4-cb840db01281\"}]},\"type\":\"ConnectorPlacement.EquallySpacedConnector\",\"uuid\":\"57d442c0-d58c-4dd4-aeba-72d113e063d7\"}],\"packageUris\":[\"http://schema.mathworks.com/mf0/Connector/19700101\"],\"version\":\"1.0\"}"
  PV4 : Subsystem
      settings: PortSchema="{\"entries\":[{\"content\":{\"sides\":[{\"content\":{\"connectorIds\":[\"In1\"]},\"type\":\"ConnectorPlacement.EquallySpacedRectSide\",\"uuid\":\"5c508248-bd07-48d5-951d-be180bcc8740\"},{\"content\":{\"connectorIds\":[],\"side\":\"RIGHT\"},\"type\":\"ConnectorPlacement.EquallySpacedRectSide\",\"uuid\":\"e31a9bdc-b533-497f-8610-a92a4eef02bc\"},{\"content\":{\"connectorIds\":[\"LConn1\"],\"side\":\"TOP\"},\"type\":\"ConnectorPlacement.EquallySpacedRectSide\",\"uuid\":\"a80efd6c-0c74-41ec-a161-3d709011a457\"},{\"content\":{\"connectorIds\":[\"RConn1\"],\"side\":\"BOTTOM\"},\"type\":\"ConnectorPlacement.EquallySpacedRectSide\",\"uuid\":\"e2d028a7-872a-45fc-84e4-cb840db01281\"}]},\"type\":\"ConnectorPlacement.EquallySpacedConnector\",\"uuid\":\"57d442c0-d58c-4dd4-aeba-72d113e063d7\"}],\"packageUris\":[\"http://schema.mathworks.com/mf0/Connector/19700101\"],\"version\":\"1.0\"}"
  + : PMIOPort  Side=Left
  - : PMIOPort  Port=2  Side=Right
  wires:
  Irr2/1 -> PV1/1(Irr)
  Irr/1 -> PV2/1(Irr)
  Irr1/1 -> PV4/1(Irr)
  Irr3/1 -> PV3/1(Irr)
  connections:
  PV2/LConn1 -- +/RConn1
  PV4/RConn1 -- PV1/LConn1
  PV4/LConn1 -- PV2/RConn1
  PV3/RConn1 -- -/RConn1
  PV1/RConn1 -- PV3/LConn1
